simulink model "simldisk2"  (R2016a)
settings: Solver=VariableStepAuto  StartTime=0.0  StopTime=10.0  RelTol=1e-3
values from neighbouring files (symbols this model uses):
  Ac = eval(subs(Alin,[x1 x2 x3 x4 u],[xlin ulin]))    [linearizacia.m]    (also in linearnySM.mat = [0 0 0 0 1 0 0 0 0 -1.962 0 -58.86 ... (16 elements, 4x4)]; linearnySM2.mat = [0 0 0 0 1 0 0 0 0 -1.962 0 58.86 ... (16 elements, 4x4)]; sysd.mat = [0 0 0 0 1 0 0 0 0 -1.962 0 -58.86 ... (16 elements, 4x4)]; sysd2.mat = [0 0 0 0 1 0 0 0 0 -1.962 0 58.86 ... (16 elements, 4x4)])
  Bc = eval(subs(Blin,[x1 x2 x3 x4 u],[xlin ulin]))    [linearizacia.m]    (also in linearnySM.mat = [0 2.5 0 12.5]; linearnySM2.mat = [0 2.5 0 -12.5]; sysd.mat = [0 2.5 0 12.5]; sysd2.mat = [0 2.5 0 -12.5])
  Cc = eval(subs(Clin,[x1 x2 x3 x4],xlin))    [linearizacia.m]    (also in linearnySM.mat = [1  0  0  0; 0  0  1  0]; linearnySM2.mat = [1  0  0  0; 0  0  1  0]; sysd.mat = [1  0  0  0; 0  0  1  0]; sysd2.mat = [1  0  0  0; 0  0  1  0])
  Dc = eval(subs(Dlin,[x1 x2 x3 x4],xlin))    [linearizacia.m]    (also in linearnySM.mat = [0 0]; linearnySM2.mat = [0 0]; sysd.mat = [0 0]; sysd2.mat = [0 0])
  dx0 = x0-xlin    [kalmankyvadlo.m]    (also in simEKFkyvadlo.m; simKFkyvadlo.m = zeros(nx,1); simdiskkyvadlo.m = [0;0;0;0]; simlinkyvadlo.m = [0;0;-pi/6;0])
settings Model: Creator=gulan  LastModifiedBy=gulan

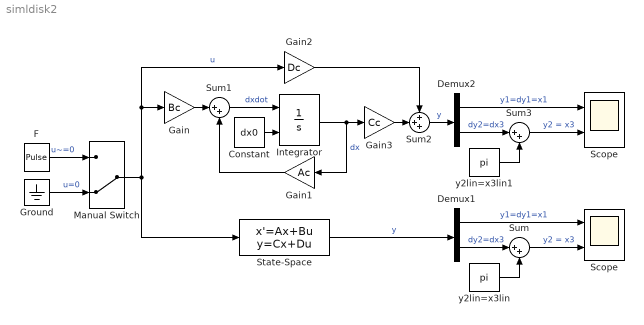
== system simldisk2 ==
  " Scope" : Scope  NumInputPorts=2
  " Scope " : Scope  NumInputPorts=2
  Constant : Constant  Value=dx0  SampleTime=0.01
  Demux1 : Demux  Outputs=2
  Demux2 : Demux  Outputs=2
  F : DiscretePulseGenerator  PulseType=Time based  Amplitude=-1  Period=10  PulseWidth=0.1  PhaseDelay=0.01
  Gain : Gain  Gain=Bc
  Gain1 : Gain  Gain=Ac
  Gain2 : Gain  Gain=Dc
  Gain3 : Gain  Gain=Cc
  Ground : Ground
  Integrator : Integrator  InitialConditionSource=external
  Manual Switch : ManualSwitch  CurrentSetting=0
  State-Space : StateSpace  A=Ac  B=Bc  C=Cc  D=Dc  X0=[0;0;0;0]
  Sum : Sum  Inputs=|++
  Sum1 : Sum  Inputs=|++
  Sum2 : Sum  Inputs=+++
  Sum3 : Sum  Inputs=|++
  y2lin=x3lin : Constant  Value=pi
  y2lin=x3lin1 : Constant  Value=pi
  wires:
  F/1 -> Manual Switch/1  "u~=0"
  Manual Switch/1 -> Gain2/1, Gain/1, State-Space/1  "u"
  Demux1/1 -> " Scope"/1  "y1=dy1=x1"
  Demux1/2 -> Sum/1  "dy2=dx3"
  Sum/1 -> " Scope"/2  "y2 = x3"
  y2lin=x3lin/1 -> Sum/2
  Gain1/1 -> Sum1/2
  Gain/1 -> Sum1/1
  Sum1/1 -> Integrator/1  "dxdot"
  Constant/1 -> Integrator/2
  Integrator/1 -> Gain3/1, Gain1/1  "dx"
  Gain2/1 -> Sum2/1
  Gain3/1 -> Sum2/2
  Demux2/1 -> " Scope "/1  "y1=dy1=x1"
  Demux2/2 -> Sum3/1  "dy2=dx3"
  Sum3/1 -> " Scope "/2  "y2 = x3"
  y2lin=x3lin1/1 -> Sum3/2
  Sum2/1 -> Demux2/1  "y"
  Ground/1 -> Manual Switch/2  "u=0"
  State-Space/1 -> Demux1/1  "y"
